simulink model "braking_without_ABS"  (R2023a)
settings: Solver=VariableStepAuto  StartTime=0.0  StopTime=20  RelTol=1e-3
libraries: simulink x2
settings Model: Creator=siddh  LastModifiedBy=siddh

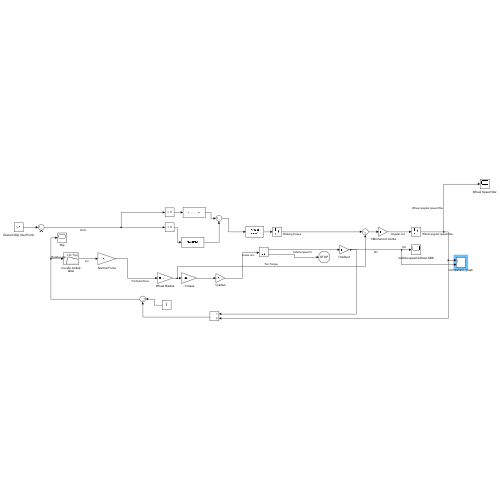
[thumbnail: Simulink's stored preview of the top-level diagram]
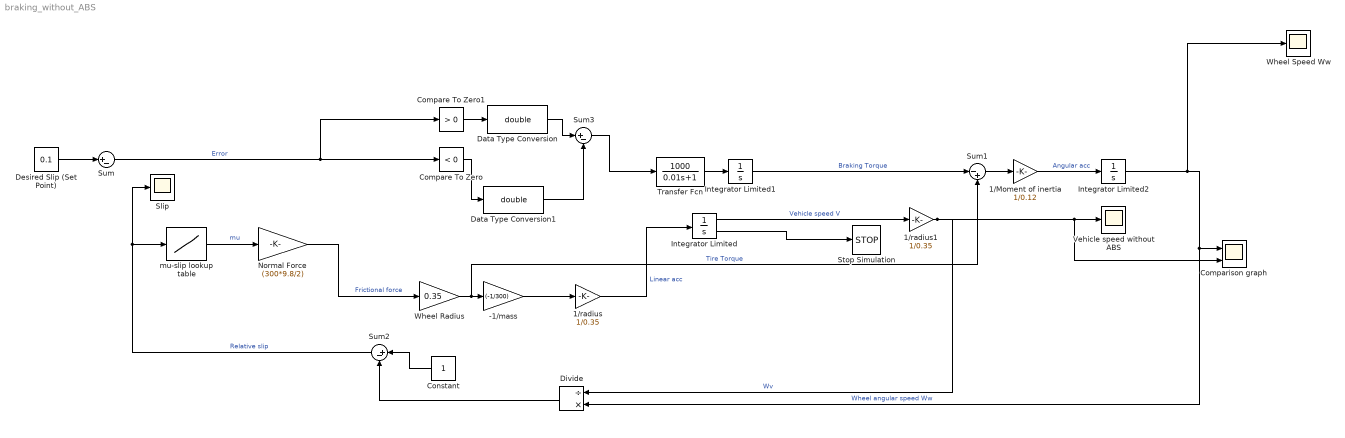
== system braking_without_ABS ==
  -1/mass : Gain  Gain=(-1/300)
  1/Moment of inertia : Gain  Gain=1/0.12
  1/radius : Gain  Gain=1/0.35
  1/radius1 : Gain  Gain=1/0.35
  Compare To Zero : simulink/Logic and Bit Operations/Compare To Zero  relop=<  OutDataTypeStr=boolean
  Compare To Zero1 : simulink/Logic and Bit Operations/Compare To Zero  relop=>  OutDataTypeStr=boolean
  Comparison graph : Scope  NumInputPorts=2
  Constant : Constant
  Data Type Conversion : DataTypeConversion  OutDataTypeStr=double  SaturateOnIntegerOverflow=off
  Data Type Conversion1 : DataTypeConversion  OutDataTypeStr=double  SaturateOnIntegerOverflow=off
  "Desired Slip (Set Point) " : Constant  Value=0.1
  Divide : Product  Inputs=/*
  Integrator Limited : Integrator  InitialCondition=30  LimitOutput=on  UpperSaturationLimit=500  LowerSaturationLimit=0  ShowSaturationPort=on
  Integrator Limited1 : Integrator  LimitOutput=on  UpperSaturationLimit=2000  LowerSaturationLimit=0
  Integrator Limited2 : Integrator  InitialCondition=30/0.35  LimitOutput=on  UpperSaturationLimit=500  LowerSaturationLimit=0
  Normal Force : Gain  Gain=(300*9.8/2)
  "Slip " : Scope
  Stop Simulation : Stop
  Sum : Sum  Inputs=|+-
  Sum1 : Sum  Inputs=|-+
  Sum2 : Sum  Inputs=|+-
  Sum3 : Sum  Inputs=|+-
  Transfer Fcn : TransferFcn  Numerator=[1000]  Denominator=[0.01 1]
  Vehicle speed without ABS : Scope
  Wheel Radius : Gain  Gain=0.35
  Wheel Speed Ww : Scope
  mu-slip lookup table : Lookup_n-D  NumberOfTableDimensions=1  BreakpointsForDimension1=[0,0.05,0.1,0.15,0.2,0.25,0.3,0.35,0.4,0.45,0.5,0.55,0.60,0.65,0.70,0.75,0.80,0.85,0.90,0.95,1]  Table=[0,0.4,0.8,0.97,1,0.98,0.96,0.94,0.92,0.9,0.88,0.855,0.83,0.81,0.79,0.77,0.75,0.73,0.72,0.71,0.7]  InternalRulePriority=Speed  RndMeth=Simplest
  wires:
  1/radius1/1 -> Divide/1, Comparison graph/2, Vehicle speed without ABS/1  "Wv"
  Sum3/1 -> Transfer Fcn/1
  Compare To Zero1/1 -> Data Type Conversion/1
  Compare To Zero/1 -> Data Type Conversion1/1
  Divide/1 -> Sum2/2
  1/Moment of inertia/1 -> Integrator Limited2/1  "Angular acc"
  Constant/1 -> Sum2/1
  Sum1/1 -> 1/Moment of inertia/1
  Transfer Fcn/1 -> Integrator Limited1/1
  1/radius/1 -> Integrator Limited/1  "Linear acc"
  Integrator Limited1/1 -> Sum1/1  "Braking Torque"
  Data Type Conversion1/1 -> Sum3/2
  Sum/1 -> Compare To Zero/1, Compare To Zero1/1  "Error"
  Integrator Limited2/1 -> Divide/2, Comparison graph/1, Wheel Speed Ww/1  "Wheel angular speed Ww"
  Integrator Limited/1 -> 1/radius1/1  "Vehicle speed V"
  "Desired Slip (Set Point) "/1 -> Sum/1
  Integrator Limited/2 -> Stop Simulation/1
  Normal Force/1 -> Wheel Radius/1  "Frictional force"
  Sum2/1 -> "Slip "/1, mu-slip lookup table/1  "Relative slip"
  mu-slip lookup table/1 -> Normal Force/1  "mu"
  -1/mass/1 -> 1/radius/1
  Wheel Radius/1 -> Sum1/2, -1/mass/1  "Tire Torque"
  Data Type Conversion/1 -> Sum3/1
